simulink model "vm_final"  (R2019b)
settings: Solver=FixedStepAuto  StartTime=0.0  StopTime=Inf  FixedStep=1e-3  RelTol=1e-3  EnableMultiTasking=on
undefined symbols (not defined in the file): D0, D1, D10, D11, D12, D13, D2, D3, D5, D6, D8, D9, PTA0, PTA1, PTA2, PTB9, PTC16, PTC17, PTC2, PTC4, PTD0, PTD1, PTD2, PTD3
libraries: frdmk64flib x27, nucleoutilitieslib x2, simulink x2, dspstat3 x1
settings Model: ExtModeTrigDuration=5  Creator=anz8  LastModifiedBy=Allen An
settings DataIOCC: ReturnWorkspaceOutputs=off
settings OptimizationCC: PassReuseOutputArgsThreshold=0  MaxStackSize=64
settings DebuggingCC: ParameterTunabilityLossMsg=error  ArithmeticOperatorsInVariantConditions=warning
settings HardwareCC: ProdBitPerPointer=32  ProdBitPerSizeT=32  ProdBitPerPtrDiffT=32  ProdLargestAtomicInteger=Long  ProdLargestAtomicFloat=Double  ProdWordSize=32  ProdHWDeviceType=ARM Compatible->ARM Cortex  UseEmbeddedCoderFeatures=off
settings SFSimCC: SimUseLocalCustomCode=off  MATLABDynamicMemAlloc=off  CustomCodeUndefinedFunction=UseInterfaceOnly
settings RTWCC: SystemTargetFile=ert.tlc  HardwareBoard=NXP FRDM-K64F  TLCOptions="-aInlineSetEventsForThisBaseRateFcn=TLC_FALSE -aSuppressMultiTaskScheduler=TLC_FALSE  -aRateBasedStepFcn=0"  TemplateMakefile=ert_default_tmf  GenerateReport=on  RTWUseLocalCustomCode=off  Toolchain=GNU Tools for ARM Embedded Processors  LaunchReport=on
settings CodeAppCC: ForceParamTrailComments=on  OperatorAnnotations=on
settings ERTTargetCC: ERTCustomFileBanners=off  SupportContinuousTime=on  SupportNonInlinedSFcns=on  RemoveResetFunc=off  ModelStepFunctionPrototypeControlCompliant=off

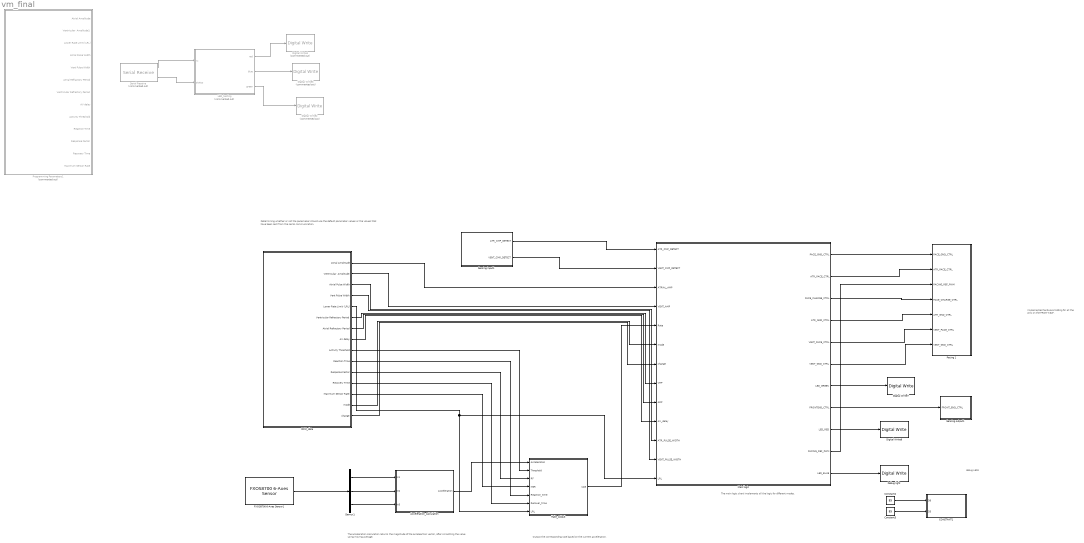
== system vm_final ==
  note: Output the corresponding rate based on the current acceleration.
  note: The acceleration calculation returns the magnitude of the acceleartion vector,
      | after smoothing the value using moving average.
  note: The main logic chart implements all the logic for different modes.
  note: debug LEDs
  note: Implemented hardware hidding for all the pins on the FRDM-K64F.
  note: Determining whether or not the pacemaker
      | should use the default parameter values or the values that
      | have been sent from the serial communication.
  Acceleration_calculation : Subsystem
  CONSTANT1 : Subsystem
  Constant2 : Constant  Value=85
  Constant3 : Constant  Value=85
  "DCM_data " : Subsystem
  Debug light : frdmk64flib/Digital Write  Whichpin=BLUE_LED
      settings: SourceProductName=Simulink Coder Support Package for NXP FRDM-K64F Board
  Demux1 : Demux  Outputs=3
  Digital Write1 : frdmk64flib/Digital Write  Commented=on  Whichpin=RED_LED
      settings: SourceProductName=Simulink Coder Support Package for NXP FRDM-K64F Board
  Digital Write2 : frdmk64flib/Digital Write  Commented=on  Whichpin=GREEN_LED
      settings: SourceProductName=Simulink Coder Support Package for NXP FRDM-K64F Board
  Digital Write3 : frdmk64flib/Digital Write  Commented=on  Whichpin=BLUE_LED
      settings: SourceProductName=Simulink Coder Support Package for NXP FRDM-K64F Board
  Digital Write7 : frdmk64flib/Digital Write  Whichpin=GREEN_LED
      settings: SourceProductName=Simulink Coder Support Package for NXP FRDM-K64F Board
  Digital Write9 : frdmk64flib/Digital Write  Whichpin=RED_LED
      settings: SourceProductName=Simulink Coder Support Package for NXP FRDM-K64F Board
  FXOS8700 6-Axes Sensor1 : frdmk64flib/FXOS8700 6-Axes Sensor  Activesensor=Accelerometer only  ODR=800Hz  HybridODR=400Hz  Accelfullrange=-4g to +4g  SampleTime=-1
      settings: SourceProductName=Simulink Coder Support Package for NXP FRDM-K64F Board
  LED_testing : Stateflow chart  Commented=on  BlockKeywords=__PRM__SERIALIZED__DATA__:Stateflow Chart,Stateflow Diagram  TreatAsAtomicUnit=on
  Main logic : Stateflow chart  TreatAsAtomicUnit=on
  Pacing 1 : Subsystem
  Programming Parameters1 : Subsystem  Commented=on
  Rate_output : Subsystem
  Sensing input1 : Subsystem
  Sensing output1 : Subsystem
  Serial Receive : frdmk64flib/Serial Receive  Commented=on  SCIModule=0  Baudrate=uint32(9600)  Parity=None  StopBits=1  HardwareFlowControl=None  ByteOrder=LittleEndian  DataType=uint8  DataLength=4  BlockingMode=off  OutputStatus=on  SampleTime=-1
      settings: SourceProductName=Simulink Coder Support Package for NXP FRDM-K64F Board
  wires:
  Demux1/3 -> Acceleration_calculation/3(In3)
  Demux1/2 -> Acceleration_calculation/2(In2)
  FXOS8700 6-Axes Sensor1/1 -> Demux1/1
  Main logic/11(LED_BLUE) -> Debug light/1
  "DCM_data "/2(Ventricular  Amplitude) -> Main logic/4(VENT_AMP)
  "DCM_data "/1("Atrial Amplitude ") -> Main logic/3(ATRIAL_AMP)
  Main logic/9(LED_RED) -> Digital Write9/1
  Main logic/8(FRONTEND_CTRL) -> Sensing output1/1(FRONT_END_CTRL)
  Sensing input1/2(VENT_CMP_DETECT) -> Main logic/2(VENT_CMP_DETECT)
  Sensing input1/1(ATR_CMP_DETECT) -> Main logic/1(ATR_CMP_DETECT)
  Constant3/1 -> CONSTANT1/2(D3)
  Constant2/1 -> CONSTANT1/1(D6)
  Main logic/7(LED_GREEN) -> Digital Write7/1
  Main logic/6(VENT_GND_CTRL) -> Pacing 1/7(VENT_GND_CTRL)
  Main logic/5(VENT_PACE_CTRL) -> Pacing 1/6(VENT_PACE_CTRL)
  Main logic/4(ATR_GND_CTRL) -> Pacing 1/5(ATR_GND_CTRL)
  Main logic/3(PACE_CHARGE_CTRL) -> Pacing 1/4(PACE_CHARGE_CTRL)
  Main logic/10(PACING_REF_PWM) -> Pacing 1/3(PACING_REF_PWM)
  Main logic/2(ATR_PACE_CTRL) -> Pacing 1/2(ATR_PACE_CTRL)
  Main logic/1(PACE_GND_CTRL) -> Pacing 1/1(PACE_GND_CTRL)
  Demux1/1 -> Acceleration_calculation/1(In1)
  LED_testing/1(red) -> Digital Write1/1
  Serial Receive/1 -> LED_testing/1(rx)
  LED_testing/2(blue) -> Digital Write3/1
  LED_testing/3(green) -> Digital Write2/1
  Serial Receive/2 -> LED_testing/2(status)
  "DCM_data "/11(Response Factor) -> Rate_output/3(RF)
  "DCM_data "/13(" Maximum Sensor Rate") -> Rate_output/4(MSR)
  "DCM_data "/12(Recovery Time) -> Rate_output/6(Recover_time)
  Acceleration_calculation/1(Acceleration) -> Rate_output/1(Acceleration)
  Rate_output/1(rate) -> Main logic/5(Rate)
  "DCM_data "/14(mode) -> Main logic/6(mode)
  "DCM_data "/9(Activity Threshold) -> Rate_output/2(Threshold)
  "DCM_data "/10(Reaction Time) -> Rate_output/5(Reaction_time)
  "DCM_data "/15(change) -> Main logic/7(change)
  "DCM_data "/8(AV delay) -> Main logic/10(AV_delay)
  "DCM_data "/6(Ventricular Refractory Period) -> Main logic/8(VRP)
  "DCM_data "/7(Atrial Refractory Period) -> Main logic/9(ARP)
  "DCM_data "/4(Vent Pulse Width) -> Main logic/12(VENT_PULSE_WIDTH)
  "DCM_data "/3(Atrial Pulse Width) -> Main logic/11(ATR_PULSE_WIDTH)
  "DCM_data "/5(Lower Rate Limit (LRL)) -> Main logic/13(LRL), Rate_output/7(LRL)

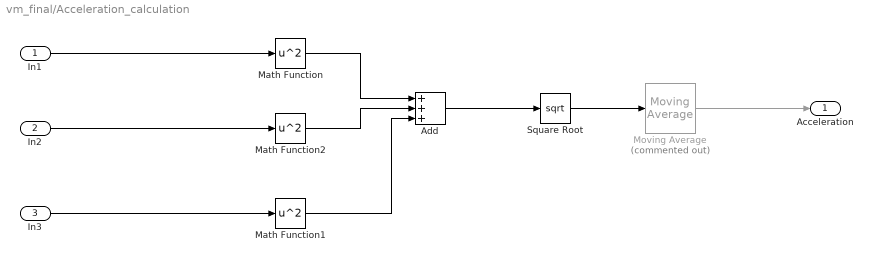
== system vm_final/Acceleration_calculation ==
  In1 : Inport
  In2 : Inport  Port=2
  In3 : Inport  Port=3
  Add : Sum  Inputs=+++
  Math Function : Math  Operator=square  SignedPower=off  SaturateOnIntegerOverflow=on
  Math Function1 : Math  Operator=square  SignedPower=off  SaturateOnIntegerOverflow=on
  Math Function2 : Math  Operator=square  SignedPower=off  SaturateOnIntegerOverflow=on
  Moving Average : dspstat3/Moving Average  Commented=on  Method=Sliding window  ForgettingFactorPort=off  SpecifyWindowLength=on  WindowLength=100  ForgettingFactor=0.9  SimulateUsing=Code generation
  Square Root : Sqrt  SaturateOnIntegerOverflow=on
  Acceleration : Outport
  wires:
  Add/1 -> Square Root/1
  Math Function1/1 -> Add/3
  Math Function2/1 -> Add/2
  Math Function/1 -> Add/1
  In3/1 -> Math Function1/1
  In2/1 -> Math Function2/1
  In1/1 -> Math Function/1
  Square Root/1 -> Moving Average/1
  Moving Average/1 -> Acceleration/1

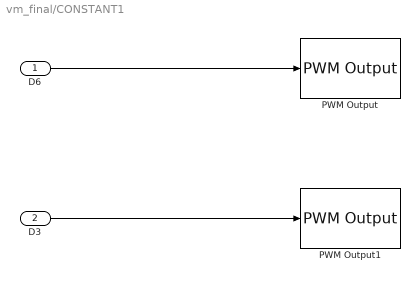
== system vm_final/CONSTANT1 ==
  D6 : Inport
  D3 : Inport  Port=2
  PWM Output : frdmk64flib/PWM Output  Whichpin=PTC2 (D6)  InitialFrequency=2000  InitialDutyCycle=75
      settings: SourceProductName=Simulink Coder Support Package for NXP FRDM-K64F Board
  PWM Output1 : frdmk64flib/PWM Output  Whichpin=PTA1 (D3)  InitialFrequency=2000  InitialDutyCycle=100
      settings: SourceProductName=Simulink Coder Support Package for NXP FRDM-K64F Board
  wires:
  D3/1 -> PWM Output1/1
  D6/1 -> PWM Output/1

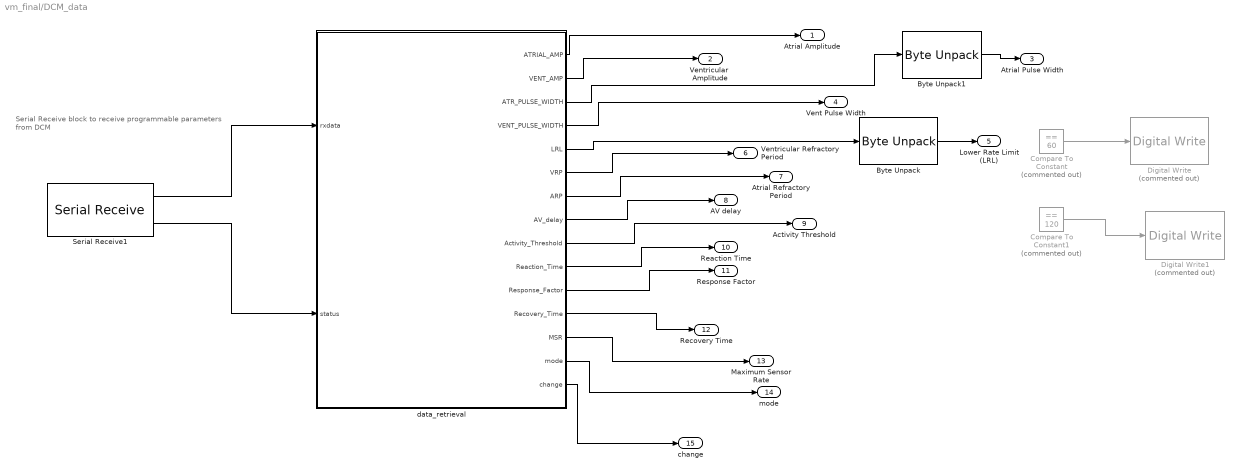
== system vm_final/DCM_data  ==
  note: Serial Receive block to receive
      | programmable parameters from DCM
  Byte Unpack : nucleoutilitieslib/Byte Unpack  dimensions={[1]}  datatypes={'uint16'}  byteAlign=1  blockPlatform=nucleo
      settings: SourceProductName=Simulink Coder Support Package for STMicroelectronics Nucleo Boards  SourceProductBaseCode=NUCLEO
  Byte Unpack1 : nucleoutilitieslib/Byte Unpack  dimensions={[1]}  datatypes={'uint16'}  byteAlign=1  blockPlatform=nucleo
      settings: SourceProductName=Simulink Coder Support Package for STMicroelectronics Nucleo Boards  SourceProductBaseCode=NUCLEO
  Compare To Constant : simulink/Logic and Bit Operations/Compare To Constant  Commented=on  relop===  const=60  OutDataTypeStr=boolean
  Compare To Constant1 : simulink/Logic and Bit Operations/Compare To Constant  Commented=on  relop===  const=120  OutDataTypeStr=boolean
  Digital Write : frdmk64flib/Digital Write  Commented=on  Whichpin=RED_LED
      settings: SourceProductName=Simulink Coder Support Package for NXP FRDM-K64F Board
  Digital Write1 : frdmk64flib/Digital Write  Commented=on  Whichpin=GREEN_LED
      settings: SourceProductName=Simulink Coder Support Package for NXP FRDM-K64F Board
  Serial Receive1 : frdmk64flib/Serial Receive  SCIModule=0  Baudrate=uint32(9600)  Parity=None  StopBits=1  HardwareFlowControl=None  ByteOrder=LittleEndian  DataType=uint8  DataLength=27  BlockingMode=off  OutputStatus=on  SampleTime=-1
      settings: SourceProductName=Simulink Coder Support Package for NXP FRDM-K64F Board
  data_retrieval : Stateflow chart  BlockKeywords=__PRM__SERIALIZED__DATA__:Stateflow Chart,Stateflow Diagram  TreatAsAtomicUnit=on
  "Atrial Amplitude " : Outport
  Ventricular  Amplitude : Outport  Port=2
  Atrial Pulse Width : Outport  Port=3
  Vent Pulse Width : Outport  Port=4
  Lower Rate Limit (LRL) : Outport  Port=5
  Ventricular Refractory Period : Outport  Port=6
  Atrial Refractory Period : Outport  Port=7
  AV delay : Outport  Port=8
  Activity Threshold : Outport  Port=9
  Reaction Time : Outport  Port=10
  Response Factor : Outport  Port=11
  Recovery Time : Outport  Port=12
  " Maximum Sensor Rate" : Outport  Port=13
  mode : Outport  Port=14
  change : Outport  Port=15
  wires:
  data_retrieval/1(ATRIAL_AMP) -> "Atrial Amplitude "/1
  Serial Receive1/1 -> data_retrieval/1(rxdata)
  Serial Receive1/2 -> data_retrieval/2(status)
  data_retrieval/7(ARP) -> Atrial Refractory Period/1
  data_retrieval/6(VRP) -> Ventricular Refractory Period/1
  data_retrieval/8(AV_delay) -> AV delay/1
  data_retrieval/9(Activity_Threshold) -> Activity Threshold/1
  data_retrieval/10(Reaction_Time) -> Reaction Time/1
  data_retrieval/11(Response_Factor) -> Response Factor/1
  data_retrieval/12(Recovery_Time) -> Recovery Time/1
  data_retrieval/13(MSR) -> " Maximum Sensor Rate"/1
  data_retrieval/2(VENT_AMP) -> Ventricular  Amplitude/1
  data_retrieval/3(ATR_PULSE_WIDTH) -> Byte Unpack1/1
  data_retrieval/4(VENT_PULSE_WIDTH) -> Vent Pulse Width/1
  data_retrieval/14(mode) -> mode/1
  data_retrieval/15(change) -> change/1
  Compare To Constant/1 -> Digital Write/1
  Compare To Constant1/1 -> Digital Write1/1
  data_retrieval/5(LRL) -> Byte Unpack/1
  Byte Unpack/1 -> Lower Rate Limit (LRL)/1
  Byte Unpack1/1 -> Atrial Pulse Width/1

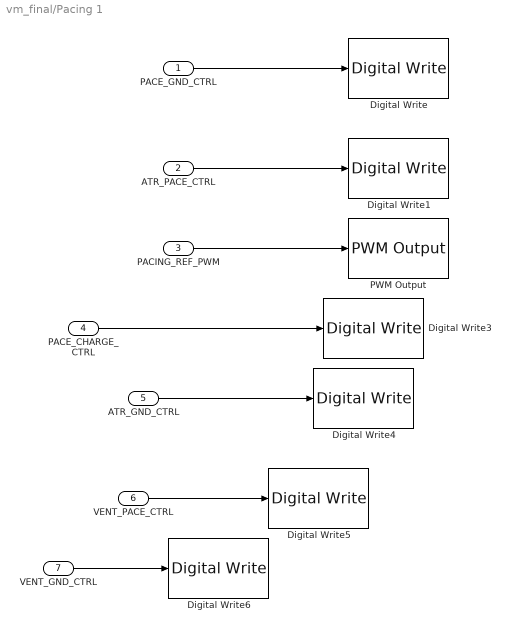
== system vm_final/Pacing 1 ==
  PACE_GND_CTRL : Inport
  ATR_PACE_CTRL : Inport  Port=2
  PACING_REF_PWM : Inport  Port=3
  PACE_CHARGE_CTRL : Inport  Port=4
  ATR_GND_CTRL : Inport  Port=5
  VENT_PACE_CTRL : Inport  Port=6
  VENT_GND_CTRL : Inport  Port=7
  Digital Write : frdmk64flib/Digital Write  Whichpin=PTD0 (D10)
      settings: SourceProductName=Simulink Coder Support Package for NXP FRDM-K64F Board
  Digital Write1 : frdmk64flib/Digital Write  Whichpin=PTA0 (D8)
      settings: SourceProductName=Simulink Coder Support Package for NXP FRDM-K64F Board
  Digital Write3 : frdmk64flib/Digital Write  Whichpin=PTB9 (D2)
      settings: SourceProductName=Simulink Coder Support Package for NXP FRDM-K64F Board
  Digital Write4 : frdmk64flib/Digital Write  Whichpin=PTD2 (D11)
      settings: SourceProductName=Simulink Coder Support Package for NXP FRDM-K64F Board
  Digital Write5 : frdmk64flib/Digital Write  Whichpin=PTC4 (D9)
      settings: SourceProductName=Simulink Coder Support Package for NXP FRDM-K64F Board
  Digital Write6 : frdmk64flib/Digital Write  Whichpin=PTD3 (D12)
      settings: SourceProductName=Simulink Coder Support Package for NXP FRDM-K64F Board
  PWM Output : frdmk64flib/PWM Output  Whichpin=PTA2 (D5)  InitialFrequency=2000  InitialDutyCycle=100
      settings: SourceProductName=Simulink Coder Support Package for NXP FRDM-K64F Board
  wires:
  VENT_GND_CTRL/1 -> Digital Write6/1
  VENT_PACE_CTRL/1 -> Digital Write5/1
  ATR_GND_CTRL/1 -> Digital Write4/1
  PACE_CHARGE_CTRL/1 -> Digital Write3/1
  PACING_REF_PWM/1 -> PWM Output/1
  ATR_PACE_CTRL/1 -> Digital Write1/1
  PACE_GND_CTRL/1 -> Digital Write/1

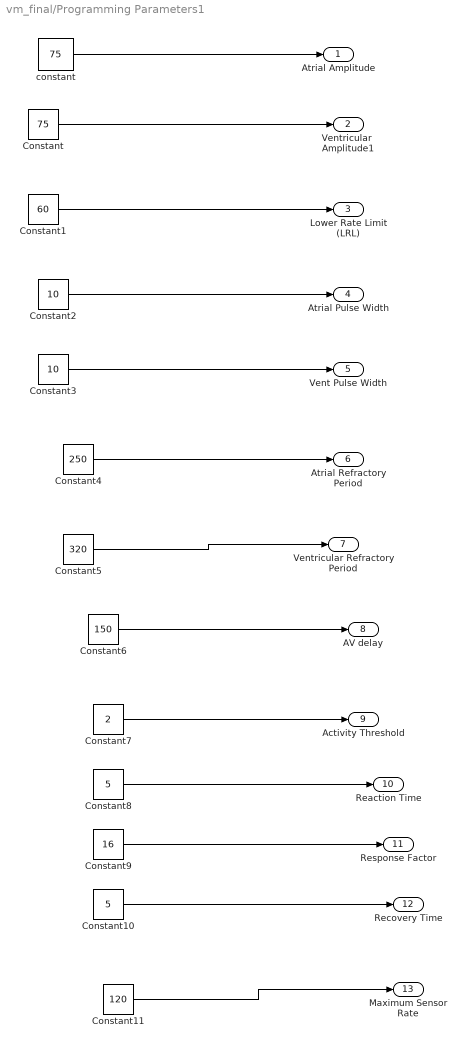
== system vm_final/Programming Parameters1 ==
  Constant : Constant  Value=75
  Constant1 : Constant  Value=60
  Constant10 : Constant  Value=5  OutDataTypeStr=double
  Constant11 : Constant  Value=120  OutDataTypeStr=double
  Constant2 : Constant  Value=10
  Constant3 : Constant  Value=10
  Constant4 : Constant  Value=250
  Constant5 : Constant  Value=320
  Constant6 : Constant  Value=150
  Constant7 : Constant  Value=2  OutDataTypeStr=double
  Constant8 : Constant  Value=5  OutDataTypeStr=double
  Constant9 : Constant  Value=16  OutDataTypeStr=double
  "constant " : Constant  Value=75
  Atrial Amplitude : Outport
  Ventricular  Amplitude1 : Outport  Port=2
  Lower Rate Limit (LRL) : Outport  Port=3
  Atrial Pulse Width : Outport  Port=4
  Vent Pulse Width : Outport  Port=5
  Atrial Refractory Period : Outport  Port=6
  Ventricular Refractory Period : Outport  Port=7
  AV delay : Outport  Port=8
  Activity Threshold : Outport  Port=9
  Reaction Time : Outport  Port=10
  Response Factor : Outport  Port=11
  Recovery Time : Outport  Port=12
  " Maximum Sensor Rate" : Outport  Port=13
  wires:
  Constant11/1 -> " Maximum Sensor Rate"/1
  Constant10/1 -> Recovery Time/1
  Constant9/1 -> Response Factor/1
  Constant8/1 -> Reaction Time/1
  Constant7/1 -> Activity Threshold/1
  Constant6/1 -> AV delay/1
  Constant5/1 -> Ventricular Refractory Period/1
  Constant3/1 -> Vent Pulse Width/1
  Constant4/1 -> Atrial Refractory Period/1
  Constant2/1 -> Atrial Pulse Width/1
  Constant1/1 -> Lower Rate Limit (LRL)/1
  Constant/1 -> Ventricular  Amplitude1/1
  "constant "/1 -> Atrial Amplitude/1

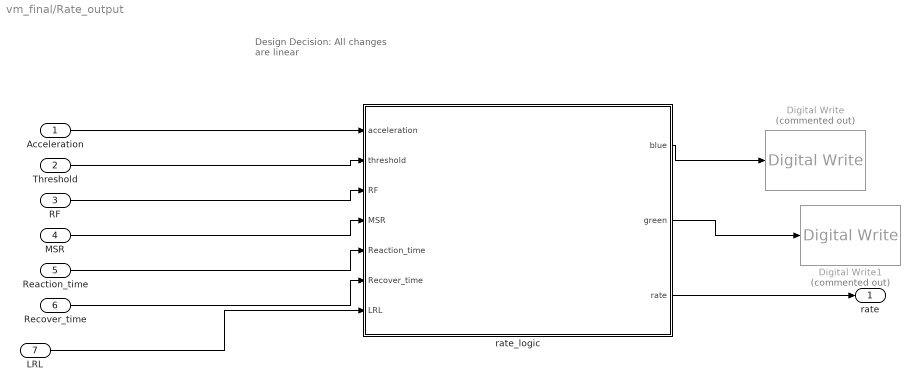
== system vm_final/Rate_output ==
  note: Design Decision:
      | All changes are linear
  Acceleration : Inport
  Threshold : Inport  Port=2
  RF : Inport  Port=3
  MSR : Inport  Port=4
  Reaction_time : Inport  Port=5
  Recover_time : Inport  Port=6
  LRL : Inport  Port=7
  Digital Write : frdmk64flib/Digital Write  Commented=on  Whichpin=BLUE_LED
      settings: SourceProductName=Simulink Coder Support Package for NXP FRDM-K64F Board
  Digital Write1 : frdmk64flib/Digital Write  Commented=on  Whichpin=GREEN_LED
      settings: SourceProductName=Simulink Coder Support Package for NXP FRDM-K64F Board
  rate_logic : Stateflow chart  BlockKeywords=__PRM__SERIALIZED__DATA__:Stateflow Chart,Stateflow Diagram  TreatAsAtomicUnit=on
  rate : Outport
  wires:
  Acceleration/1 -> rate_logic/1(acceleration)
  Threshold/1 -> rate_logic/2(threshold)
  RF/1 -> rate_logic/3(RF)
  MSR/1 -> rate_logic/4(MSR)
  Reaction_time/1 -> rate_logic/5(Reaction_time)
  Recover_time/1 -> rate_logic/6(Recover_time)
  rate_logic/1(blue) -> Digital Write/1
  rate_logic/2(green) -> Digital Write1/1
  rate_logic/3(rate) -> rate/1
  LRL/1 -> rate_logic/7(LRL)

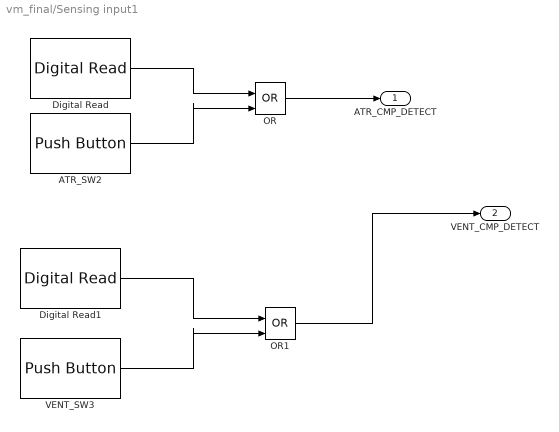
== system vm_final/Sensing input1 ==
  ATR_SW2 : frdmk64flib/Push Button  Whichswitch=SW2  SampleTime1=-1
      settings: SourceProductName=Simulink Coder Support Package for NXP FRDM-K64F Board
  Digital Read : frdmk64flib/Digital Read  Whichpin=PTC16 (D0)  SampleTime=-1
      settings: SourceProductName=Simulink Coder Support Package for NXP FRDM-K64F Board
  Digital Read1 : frdmk64flib/Digital Read  Whichpin=PTC17 (D1)  SampleTime=-1
      settings: SourceProductName=Simulink Coder Support Package for NXP FRDM-K64F Board
  OR : Logic  Operator=OR  IconShape=distinctive  AllPortsSameDT=off  OutDataTypeStr=boolean
  OR1 : Logic  Operator=OR  IconShape=distinctive  AllPortsSameDT=off  OutDataTypeStr=boolean
  VENT_SW3 : frdmk64flib/Push Button  Whichswitch=SW3  SampleTime1=-1
      settings: SourceProductName=Simulink Coder Support Package for NXP FRDM-K64F Board
  ATR_CMP_DETECT : Outport
  VENT_CMP_DETECT : Outport  Port=2
  wires:
  Digital Read/1 -> OR/1
  Digital Read1/1 -> OR1/1
  OR1/1 -> VENT_CMP_DETECT/1
  VENT_SW3/1 -> OR1/2
  ATR_SW2/1 -> OR/2
  OR/1 -> ATR_CMP_DETECT/1

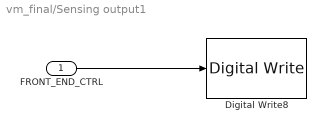
== system vm_final/Sensing output1 ==
  FRONT_END_CTRL : Inport
  Digital Write8 : frdmk64flib/Digital Write  Whichpin=PTD1 (D13)
      settings: SourceProductName=Simulink Coder Support Package for NXP FRDM-K64F Board
  wires:
  FRONT_END_CTRL/1 -> Digital Write8/1

== stateflow chart vm_final/LED_testing ==
  state IDLE_state
    red=0;
  state initial_state
    entry:
    red=0;
    green=0;
    blue=0;
  state set_led
    entry:
    red=rx(2);
    green=rx(3);
    blue=rx(4);
    %blue=1;
  set_led -> IDLE_state
  (default) -> initial_state
  initial_state -> IDLE_state
  IDLE_state -> set_led : [status==0]
  data: rx input uint8; red output uint8; blue output uint8; green output uint8; status input uint8

== stateflow chart vm_final/Main logic ==
  state AOOR
    %charge and discharge
    entry:
    VENT_PACE_CTRL=false;% turn off vent
    VENT_GND_CTRL=false;
    PACE_GND_CTRL=true; % 10 on
    ATR_PACE_CTRL=false; % 6 off
    %PACING_REF_PWM=true; %1 on
    PACING_REF_PWM=ATRIAL_AMP;
    PACE_CHARGE_CTRL=true; % 4 on
    ATR_GND_CTRL=true; % 7 on
    LED_RED=false;
    LED_GREEN=false;
  state ATRIUM_Pacing2
    entry:
    %4 off, 6 on ,7 off
    PACE_CHARGE_CTRL=false; %4 off
    ATR_PACE_CTRL=true; % 6 on
    ATR_GND_CTRL=false; % 7 off
    LED_RED=true;
  note: Mode 0 used for debugging
  state byebye
    entry:
    LED_RED=false;
    LED_BLUE=false;
    LED_GREEN=false;
  state OFFFFFFFFF
    entry:
    LED_RED=true;
    LED_BLUE=true;
    LED_GREEN=true;
  state ATRIUM_Pacing
    entry:
    %4 off, 6 on ,7 off
    PACE_CHARGE_CTRL=false; %4 off
    ATR_PACE_CTRL=true; % 6 on
    ATR_GND_CTRL=false; % 7 off
    LED_RED=true;
  state AOO
    %charge and discharge
    entry:
    VENT_PACE_CTRL=false;% turn off vent
    VENT_GND_CTRL=false;
    PACE_GND_CTRL=true; % 10 on
    ATR_PACE_CTRL=false; % 6 off
    %PACING_REF_PWM=true; %1 on
    PACING_REF_PWM=ATRIAL_AMP;
    PACE_CHARGE_CTRL=true; % 4 on
    ATR_GND_CTRL=true; % 7 on
    LED_RED=false;
    LED_GREEN=false;
  state DOO
    entry:
    %charge and discharge for AOO
    %A charging V discharging
    VENT_PACE_CTRL=false;% turn off vent
    VENT_GND_CTRL=false;
    PACE_GND_CTRL=true; % 10 on
    ATR_PACE_CTRL=false; % 6 off
    %PACING_REF_PWM=true; %1 on
    PACING_REF_PWM=ATRIAL_AMP;
    PACE_CHARGE_CTRL=true; % 4 on
    VENT_GND_CTRL=true; % 7 on
    LED_GREEN=false;
  state A_Pacing
    entry:
    %4 off, 6 on ,7 off
    PACE_CHARGE_CTRL=false; %4 off
    ATR_PACE_CTRL=true; % 6 on
    VENT_GND_CTRL=false; % 7 off
    LED_RED=true;
  state MAIN
    entry:
    LED_RED=false;
    LED_GREEN=true;
    LED_BLUE=false;
  state VENT_Pacing
    entry:
    %4 off, 6 on ,7 off
    PACE_CHARGE_CTRL=false; %4 off
    VENT_PACE_CTRL=true; % 6 on
    VENT_GND_CTRL=false; % 7 off
    LED_BLUE=true;
  state VOO
    entry:
    %charge and discharge
    ATR_PACE_CTRL=false;%turn off atrium
    ATR_GND_CTRL=false;
    PACE_GND_CTRL=true; % 10 on
    VENT_PACE_CTRL=false; % 6 off
    %PACING_REF_PWM=true; %1 on
    PACING_REF_PWM=VENT_AMP;
    PACE_CHARGE_CTRL=true; % 4 on
    VENT_GND_CTRL=true; % 7 on
    LED_BLUE=false;
    LED_GREEN=false;
  state AAI
    entry:
    FRONTEND_CTRL=true; %2 on
    LED_RED=false;
    %charge and discharge
    VENT_PACE_CTRL=false;% turn off vent
    VENT_GND_CTRL=false;
    PACE_GND_CTRL=true; % 10 on
    ATR_PACE_CTRL=false; % 6 off
    %PACING_REF_PWM=true; %1 on
    PACING_REF_PWM=ATRIAL_AMP;
    PACE_CHARGE_CTRL=true; % 4 on
    ATR_GND_CTRL=true; % 7 on
    LED_GREEN=false;
  state V_charging_A_discharging
    entry:
    %charge and discharge
    ATR_PACE_CTRL=false;%turn off atrium
    ATR_GND_CTRL=false;
    PACE_GND_CTRL=true; % 10 on
    VENT_PACE_CTRL=false; % 6 off
    %PACING_REF_PWM=true; %1 on
    PACING_REF_PWM=VENT_AMP;
    PACE_CHARGE_CTRL=true; % 4 on
    ATR_GND_CTRL=true; % 7 on
    LED_RED=false;
  state V_pacing
    entry:
    %4 off, 6 on ,7 off
    PACE_CHARGE_CTRL=false; %4 off
    VENT_PACE_CTRL=true; % 6 on
    ATR_GND_CTRL=false; % 7 off
    LED_GREEN=true;
  state ATRIUM_Pacing3
    entry:
    %4 off, 6 on ,7 off
    PACE_CHARGE_CTRL=false; %4 off
    ATR_PACE_CTRL=true; % 6 on
    ATR_GND_CTRL=false; % 7 off
    LED_GREEN=true;
    timeAAI=60/LRL*1000-ATR_PULSE_WIDTH;
  state VVI
    entry:
    FRONTEND_CTRL=true; %2 on
    LED_RED=false;
    %charge and discharge
    ATR_PACE_CTRL=false;%turn off atrium
    ATR_GND_CTRL=false;;
    PACE_GND_CTRL=true; % 10 on
    VENT_PACE_CTRL=false; % 6 off
    %PACING_REF_PWM=true; %1 on
    PACING_REF_PWM=VENT_AMP;
    PACE_CHARGE_CTRL=true; % 4 on
    VENT_GND_CTRL=true; % 7 on
    LED_GREEN=false;
  state waiting_ATR1
    entry:
    FRONTEND_CTRL=false; %2 off
    LED_RED=true;
    timeAAI=60/LRL*1000-ATR_PULSE_WIDTH-ARP;
  state VENT_Pacing2
    entry:
    %4 off, 6 on ,7 off
    PACE_CHARGE_CTRL=false; %4 off
    VENT_PACE_CTRL=true; % 6 on
    VENT_GND_CTRL=false; % 7 off
    LED_GREEN=true;
    timeVVI=60/LRL*1000-VENT_PULSE_WIDTH;
  state waiting_VENT1
    entry:
    FRONTEND_CTRL=false; %2 off
    LED_RED=true;
    timeVVI=60/LRL*1000-VENT_PULSE_WIDTH-VRP;
  AOOR -> ATRIUM_Pacing2 [order 1] : after(60*1000/Rate-ATR_PULSE_WIDTH,msec)
  ATRIUM_Pacing2 -> AOOR : after(ATR_PULSE_WIDTH,msec)
  MAIN -> AOOR [order 1] : [mode==6]
  AOOR -> MAIN [order 2] : [change==true]
  OFFFFFFFFF -> byebye : after(400,msec)
  byebye -> OFFFFFFFFF [order 2] : after(400,msec)
  byebye -> MAIN [order 1] : [change==true]
  MAIN -> byebye [order 7] : [mode==0]
  AOO -> MAIN [order 2] : [change==true]
  ATRIUM_Pacing -> AOO : after(ATR_PULSE_WIDTH,msec)
  AOO -> ATRIUM_Pacing [order 1] : after(60/LRL*1000-ATR_PULSE_WIDTH,msec)
  (default) -> MAIN
  MAIN -> AOO [order 2] : [mode==1]
  DOO -> A_Pacing [order 1] : after(60/LRL*1000-VENT_PULSE_WIDTH-AV_delay,msec)
  MAIN -> DOO [order 6] : [mode==5]
  VOO -> VENT_Pacing [order 1] : after(60/LRL*1000-VENT_PULSE_WIDTH,msec)
  DOO -> MAIN [order 2] : [change==true]
  MAIN -> VOO [order 3] : [mode==2]
  VENT_Pacing -> VOO : after(VENT_PULSE_WIDTH,msec)
  VOO -> MAIN [order 2] : [change==true]
  A_Pacing -> V_charging_A_discharging : after(ATR_PULSE_WIDTH,msec)
  VVI -> MAIN [order 2] : [change==true]
  MAIN -> VVI [order 5] : [mode==4]
  AAI -> MAIN [order 3] : [change==true]
  MAIN -> AAI [order 4] : [mode==3]
  V_pacing -> DOO : after(VENT_PULSE_WIDTH,msec)
  V_charging_A_discharging -> V_pacing : after(AV_delay-ATR_PULSE_WIDTH,msec)
  AAI -> ATRIUM_Pacing3 [order 2] : after(timeAAI,msec)
  ATRIUM_Pacing3 -> AAI : after(ATR_PULSE_WIDTH,msec)
  waiting_ATR1 -> AAI : after(ARP,msec)
  AAI -> waiting_ATR1 [order 1] : [ATR_CMP_DETECT==true]
  VVI -> VENT_Pacing2 [order 1] : after(timeVVI,msec)
  waiting_VENT1 -> VVI : after(VRP,msec)
  VVI -> waiting_VENT1 [order 3] : [VENT_CMP_DETECT==true]
  VENT_Pacing2 -> VVI : after(VENT_PULSE_WIDTH,msec)
  data: PACE_GND_CTRL output boolean; ATR_PACE_CTRL output boolean; PACE_CHARGE_CTRL output boolean; ATR_GND_CTRL output boolean; VENT_PACE_CTRL output boolean; VENT_GND_CTRL output boolean; LED_GREEN output boolean; ATR_CMP_DETECT input boolean; VENT_CMP_DETECT input boolean; FRONTEND_CTRL output boolean; LED_RED output boolean; ATRIAL_AMP input uint8; VENT_AMP input uint8; PACING_REF_PWM output uint8; LED_BLUE output boolean; Rate input uint16; mode input uint8; change input uint8; timeAAI local uint16; timeVVI local uint16; ATR_PULSE_WIDTH_IN local uint8; VENT_PULSE_WIDTH_IN local uint8; AV_delay_IN local uint8; LRL_IN local uint8; VRP input uint16; ARP input uint16; AV_delay input uint16; VRP_IN local uint16; ARP_IN local uint16; ATR_PULSE_WIDTH input uint16; VENT_PULSE_WIDTH input uint16; LRL input uint16

== stateflow chart vm_final/DCM_data /data_retrieval ==
  note: If the serial communication did not work, the default assigned values will be used.
  state SET_PARAM
    entry:
    mode= rxdata(3);
    LRL=typecast(rxdata(4:5),'uint16');
    MSR=typecast(rxdata(6:7),'uint16');
    AV_delay= typecast(rxdata(8:9),'uint16');
    ATRIAL_AMP=rxdata(10);
    VENT_AMP=rxdata(11);
    ATR_PULSE_WIDTH=typecast(rxdata(12:13),'uint16');
    VENT_PULSE_WIDTH=typecast(rxdata(14:15),'uint16');
    VRP=typecast(rxdata(16:17),'uint16');%320
    ARP=typecast(rxdata(18:19),'uint16');%250
    Activity_Threshold=typecast(rxdata(20:21),'uint16');
    Reaction_Time=typecast(rxdata(22:23),'uint16');
    Response_Factor=typecast(rxdata(24:25),'uint16');
    Recovery_Time=typecast(rxdata(26:27),'uint16');
    change=1;
  state Initial
    entry:
    mode=0;
    LRL=60; %60
    MSR=120; %120
    AV_delay= 150; %150
    ATRIAL_AMP=75; %75
    VENT_AMP=75; %75
    ATR_PULSE_WIDTH=10; %10
    VENT_PULSE_WIDTH=10; %10
    VRP=320%320
    ARP=250;%250
    Activity_Threshold=2;
    Reaction_Time=5;
    Response_Factor=10;
    Recovery_Time=5;
    change=0;
  state Standby
    %waiting for COM
    change=0;
  (default) -> Initial
  SET_PARAM -> Standby : after(2000,msec)
  Standby -> SET_PARAM : [status==0 && rxdata(1)==hex2dec('16')&&rxdata(2)==hex2dec('55')]
  Initial -> Standby
  data: rxdata input uint8; status input uint8; ATRIAL_AMP output uint8; VENT_AMP output uint8; ATR_PULSE_WIDTH output uint16; VENT_PULSE_WIDTH output uint16; LRL output uint16; VRP output uint16; ARP output uint16; AV_delay output uint16; Activity_Threshold output uint16; Reaction_Time output uint16; Response_Factor output uint16; Recovery_Time output uint16; MSR output uint16; mode output uint8; change output uint8

== stateflow chart vm_final/Rate_output/rate_logic ==
  state Initial_setup
    entry:
    green=false;
    blue=false;
    rate=LRL;
  state DOWN
    entry:
    step_down=(rate-LRL)/Recover_time;
    green=false;
  state Low
    entry:
    target_rate = 0.8*RF *(acceleration - threshold) + LRL;
    if target_rate >= MSR
    target_rate = MSR;
    end
    step_up=(target_rate-rate)/Reaction_time;
    blue=false;
  state High [commented out]
    entry:
    rate=MSR;
  state rate_decrement
    entry:
    rate=rate-step_down;
    green=true;
  state rate_increment
    entry:
    rate=rate+step_up;
    blue=true;
  (default) -> Initial_setup
  Initial_setup -> DOWN
  Low -> DOWN [order 1] : [acceleration<threshold]
  Low -> High [commented out] : [rate>=MSR]
  DOWN -> Low [order 1] : [acceleration>=threshold]
  rate_decrement -> DOWN
  DOWN -> rate_decrement [order 2] : after(1000,msec)
  High -> Low [commented out]
  Low -> rate_increment [order 2] : after(1000,msec)
  rate_increment -> Low
  data: acceleration input double; threshold input uint16; RF input uint16; MSR input uint16; Reaction_time input uint16; Recover_time input uint16; blue output boolean; green output boolean; rate output uint16; LRL input uint16; step_up local uint16; step_down local uint16; target_rate local uint16
